simulink model "gm_HDLQAMDemod_vs"  (R2024a)
settings: Solver=FixedStepDiscrete  StartTime=0.0  StopTime=stopTime  RelTol=1e-3
undefined symbols (not defined in the file or in its folder): clk, clk_enable, fs, QAM, reset_x
libraries: dspsrcs4 x3, whdlmod x3, simulink x2, whdlutilities x1, vivadosimlib x1, HDL_ieee_8021513 x1
settings Model: Creator=cotti  LastModifiedBy=cotti
settings OptimizationCC: BlockReduction=off  ConditionallyExecuteInputs=off  DefaultParameterBehavior=Inlined  InheritOutputTypeSmallerThanSingle=on
settings DebuggingCC: AlgebraicLoopMsg=error  ArtificialAlgebraicLoopMsg=error  InheritedTsInSrcMsg=none  SingleTaskRateTransMsg=error  UnconnectedInputMsg=warning  UnconnectedOutputMsg=warning  UnconnectedLineMsg=warning
settings HardwareCC: ProdBitPerPointer=32  ProdBitPerSizeT=32  ProdBitPerPtrDiffT=32  ProdLargestAtomicFloat=None  ProdIntDivRoundTo=Undefined  ProdEndianess=Unspecified  ProdWordSize=32  ProdHWDeviceType=ASIC/FPGA->ASIC/FPGA  TargetBitPerLong=64  TargetBitPerPointer=64  TargetBitPerSizeT=64  TargetBitPerPtrDiffT=64  TargetLongLongMode=on  TargetIntDivRoundTo=Zero  TargetEndianess=LittleEndian  TargetWordSize=64  TargetHWDeviceType=Custom Processor->MATLAB Host Computer  ProdEqTarget=off

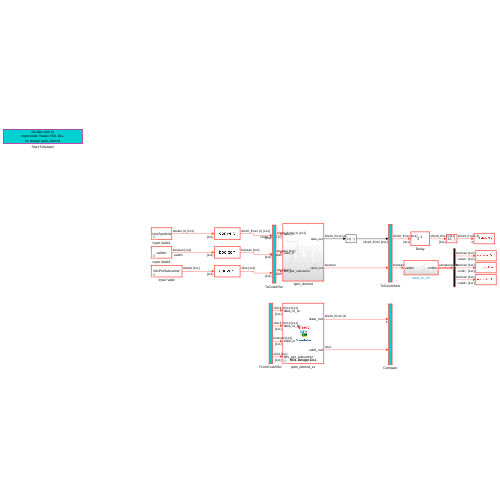
[thumbnail: Simulink's stored preview of the top-level diagram]
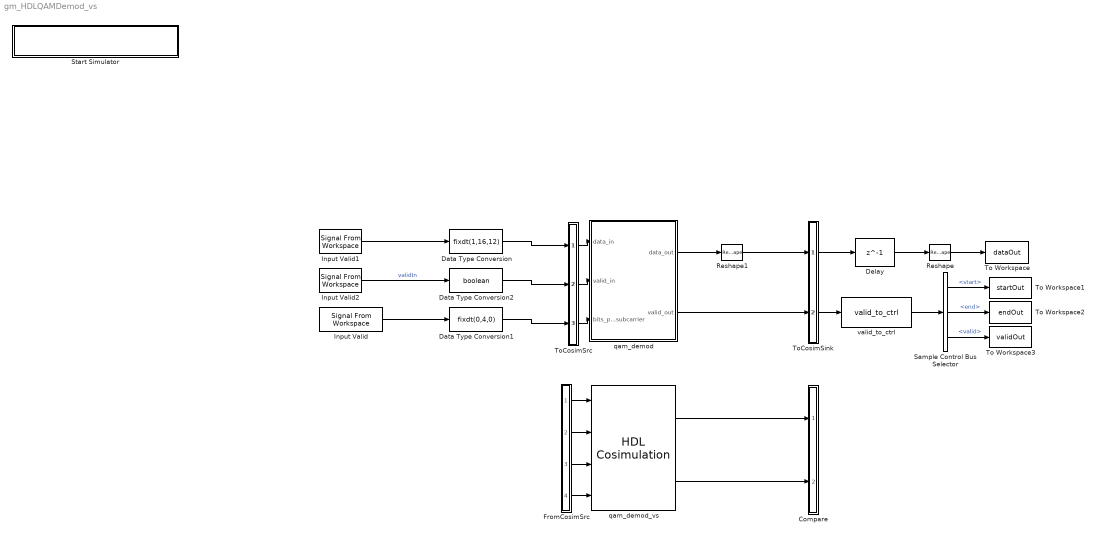
== system gm_HDLQAMDemod_vs ==
  Compare : Subsystem
      mask Display: disp('')
  Data Type Conversion : DataTypeConversion  OutDataTypeStr=fixdt(1,16,12)  SaturateOnIntegerOverflow=off  RndMeth=Floor
  Data Type Conversion1 : DataTypeConversion  OutDataTypeStr=fixdt(0,4,0)  SaturateOnIntegerOverflow=off  RndMeth=Floor
  Data Type Conversion2 : DataTypeConversion  OutDataTypeStr=boolean  SaturateOnIntegerOverflow=off  RndMeth=Floor
  Delay : Delay  DelayLength=1  InitialCondition=0  UseCircularBuffer=on
  FromCosimSrc : Subsystem
      mask Display: disp('')
  Input Valid : dspsrcs4/Signal From Workspace  X=bitsPerSubcarrier  Ts=1/fs  nsamps=1  OutputAfterFinalValue=Setting to zero  ignoreOrWarnInputAndFrameLengths=off  OutputFrames=off
  Input Valid1 : dspsrcs4/Signal From Workspace  X=dataSymbols  Ts=1/fs  nsamps=1  OutputAfterFinalValue=Setting to zero  ignoreOrWarnInputAndFrameLengths=off  OutputFrames=off
  Input Valid2 : dspsrcs4/Signal From Workspace  X=validIn  Ts=1/fs  nsamps=1  OutputAfterFinalValue=Setting to zero  ignoreOrWarnInputAndFrameLengths=off  OutputFrames=off
  Reshape : Reshape
  Reshape1 : Reshape
  Sample Control Bus Selector : whdlutilities/Sample Control Bus Selector  OutputSignals=start,end,valid
  Start Simulator : Subsystem
      settings: OpenFcn=|
      | cosimDirName = pwd;
      | cd 'hdl_prj/hdlsrc/HDLQAMDemod';
      | [s,r] = system('vivado -mode batch -source gm_HDLQAMDemod_vs.tcl','-echo');
      | cd (cosimDirName);
      | clear cosimDirName;
      | if s
      |    error('Failed to create Vivado HDL design DLL using script gm_HDLQAMDemod_vs.tcl.');
      | end
      mask Display: disp('Double-click to\nregenerate Vivado HDL DLL\nfor design qam_demod')
  To Workspace : ToWorkspace  VariableName=dataOut  SampleTime=1/fs
      settings: Save2DSignal=2-D array (concatenate along first dimension)
  To Workspace1 : ToWorkspace  VariableName=startOut  SampleTime=1/fs
      settings: Save2DSignal=2-D array (concatenate along first dimension)
  To Workspace2 : ToWorkspace  VariableName=endOut  SampleTime=1/fs
      settings: Save2DSignal=2-D array (concatenate along first dimension)
  To Workspace3 : ToWorkspace  VariableName=validOut  SampleTime=1/fs
      settings: Save2DSignal=2-D array (concatenate along first dimension)
  ToCosimSink : Subsystem
      mask Display: disp('')
  ToCosimSrc : Subsystem
      mask Display: disp('')
  qam_demod : Subsystem
  qam_demod_vs : vivadosimlib/HDL Cosimulation  PortPaths=/qam_demod/data_in_re;/qam_demod/data_in_im;/qam_demod/valid_in;/qam_demod/bits_per_subcarrier;/qam_demod/data_out;/qam_demod/valid_out  PortModes=[1 1 1 1 2 2 ]  PortTimes=[-1 -1 -1 -1 1.0000000000000000209225608301284726753266340892878361046314239502e-08 1.0000000000000000209225608301284726753266340892878361046314239502e-08 ]  PortSigns=[-1 -1 -1 -1 1 0 ]  PortFracLengths=[0,0,0,0,12,0]  PortWordLengths=[-1,-1,-1,-1,20,1]  PortHDLWordSizes=[16,16,1,4,20,1]  CommLocal=on  CommSharedMemory=on  CommPortNumber=4449  CommShowInfo=on  ClockPaths=clk;clk_enable;reset_x;  ClockModes=[2 4 3]  ClockTimes=[1e-08 3.7e-08 2.7e-08]  TclPostSimCommand="puts \"done\""  TimingMode=ns  TimingScaleFactor=1000000000  idxCellArray={'UNUSED_VAR'}  CosimBypass=Full Simulation  AllowDirectFeedthrough=on  ProductName=EDA Simulator Link VS  RunAutoTimescale=off  HdlClocks=0  PreRunTime=40  PreRunTimeUnit=ns
  valid_to_ctrl : HDL_ieee_8021513/valid_to_ctrl  SystemSampleTime=-1  VariantActivationTime=update diagram  AllowFlexibleInterface=on  Latency=0  AutoFrameSizeCalculation=off
      settings: SourceProductName=HDL IEEE 8021513
  wires:
  Sample Control Bus Selector/2 -> To Workspace2/1  "<end>"
  Input Valid/1 -> Data Type Conversion1/1
  Input Valid2/1 -> Data Type Conversion2/1  "validIn"
  Sample Control Bus Selector/3 -> To Workspace3/1  "<valid>"
  Input Valid1/1 -> Data Type Conversion/1
  valid_to_ctrl/1 -> Sample Control Bus Selector/1
  Sample Control Bus Selector/1 -> To Workspace1/1  "<start>"
  Delay/1 -> Reshape/1
  Reshape/1 -> To Workspace/1
  ToCosimSrc/1(out1) -> qam_demod/1(data_in)
  ToCosimSrc/2(out2) -> qam_demod/2(valid_in)
  ToCosimSrc/3(out3) -> qam_demod/3(bits_per_subcarrier)
  qam_demod/1(data_out) -> Reshape1/1
  qam_demod/2(valid_out) -> ToCosimSink/2(in2)
  Data Type Conversion/1 -> ToCosimSrc/1(in1)
  Data Type Conversion2/1 -> ToCosimSrc/2(in2)
  Data Type Conversion1/1 -> ToCosimSrc/3(in3)
  ToCosimSink/1(out1) -> Delay/1
  ToCosimSink/2(out2) -> valid_to_ctrl/1
  FromCosimSrc/1(out1) -> qam_demod_vs/1
  FromCosimSrc/2(out2) -> qam_demod_vs/2
  FromCosimSrc/3(out3) -> qam_demod_vs/3
  FromCosimSrc/4(out4) -> qam_demod_vs/4
  qam_demod_vs/1 -> Compare/1(in1)
  qam_demod_vs/2 -> Compare/2(in2)
  Reshape1/1 -> ToCosimSink/1(in1)

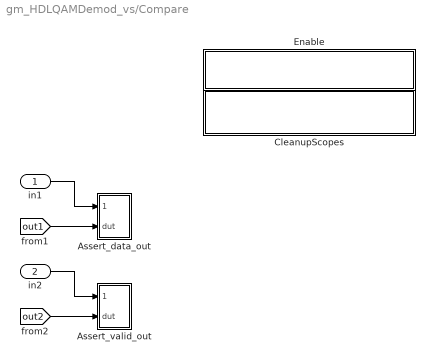
== system gm_HDLQAMDemod_vs/Compare ==
  in1 : Inport
  in2 : Inport  Port=2
  Assert_data_out : Subsystem
      settings: LibrarySourceBlock=hdlmdlgenlib/AssertEq
  Assert_valid_out : Subsystem
      settings: LibrarySourceBlock=hdlmdlgenlib/AssertEq
  CleanupScopes : Subsystem
      settings: OpenFcn=|
      | blkName = gcb; %self block
      | idx = regexp(blkName, '/CleanupScopes$', 'once');
      | blkParent = blkName(1:idx-1);
      | blks=find_system(blkParent, 'LookUnderMasks', 'all','blocktype', 'Scope');
      | for itr = 1:length(blks)
      | 	 hScopeCfg = get_param(blks{itr},'ScopeConfiguration');
      | 	 hScopeCfg.Visible = ~ hScopeCfg.Visible;
      | end
      | drawnow;
      mask Display: fprintf(message('hdlcoder:cosim:vnl_dblclick').getString());
  Enable : Subsystem
      settings: OpenFcn=|
      | blkName = gcb;
      | idx = regexp(blkName, '/Enable$', 'once');
      | blkParent = blkName(1:idx-1);
      | blks=find_system(blkParent, 'LookUnderMasks', 'all','blocktype', 'Assertion');
      | e = get_param(blks{1}, 'Enabled');
      | if strcmp(e, 'on'), f= 'off';, else, f = 'on';, end
      | for ii=1:length(blks), set_param(blks{ii}, 'Enabled', f);, end
      | set_param(gcb, 'MaskDisplay',['fprintf(message(''hdlcoder:cosim:vnl_dblclick_assertions'',','''',upper(e),'''',').getString())']);
      mask Display: fprintf(message('hdlcoder:cosim:vnl_dblclick_assertions','OFF').getString());
  wires:
  [out2] -> Assert_valid_out/2(dut)
  in2/1 -> Assert_valid_out/1(cosim)
  [out1] -> Assert_data_out/2(dut)
  in1/1 -> Assert_data_out/1(cosim)

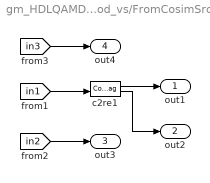
== system gm_HDLQAMDemod_vs/FromCosimSrc ==
  c2re1 : ComplexToRealImag
  out1 : Outport
  out2 : Outport  Port=2
  out3 : Outport  Port=3
  out4 : Outport  Port=4
  wires:
  c2re1/2 -> out2/1
  [in2] -> out3/1
  [in1] -> c2re1/1
  c2re1/1 -> out1/1
  [in3] -> out4/1

== system gm_HDLQAMDemod_vs/Start Simulator ==

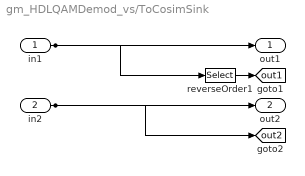
== system gm_HDLQAMDemod_vs/ToCosimSink ==
  in1 : Inport
  in2 : Inport  Port=2
  reverseOrder1 : Selector  IndexOptions=Index vector (dialog)  Indices=[4:-1:1]  OutputSizes=1
  out1 : Outport
  out2 : Outport  Port=2
  tag scope: out1=global, out2=global
  wires:
  in1/1 -> out1/1, reverseOrder1/1
  reverseOrder1/1 -> [out1]
  in2/1 -> out2/1, [out2]

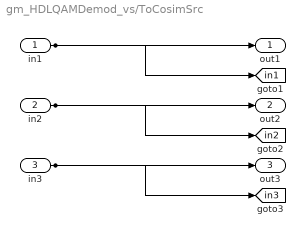
== system gm_HDLQAMDemod_vs/ToCosimSrc ==
  in1 : Inport
  in2 : Inport  Port=2
  in3 : Inport  Port=3
  out1 : Outport
  out2 : Outport  Port=2
  out3 : Outport  Port=3
  tag scope: in1=global, in2=global, in3=global
  wires:
  in1/1 -> out1/1, [in1]
  in2/1 -> out2/1, [in2]
  in3/1 -> out3/1, [in3]

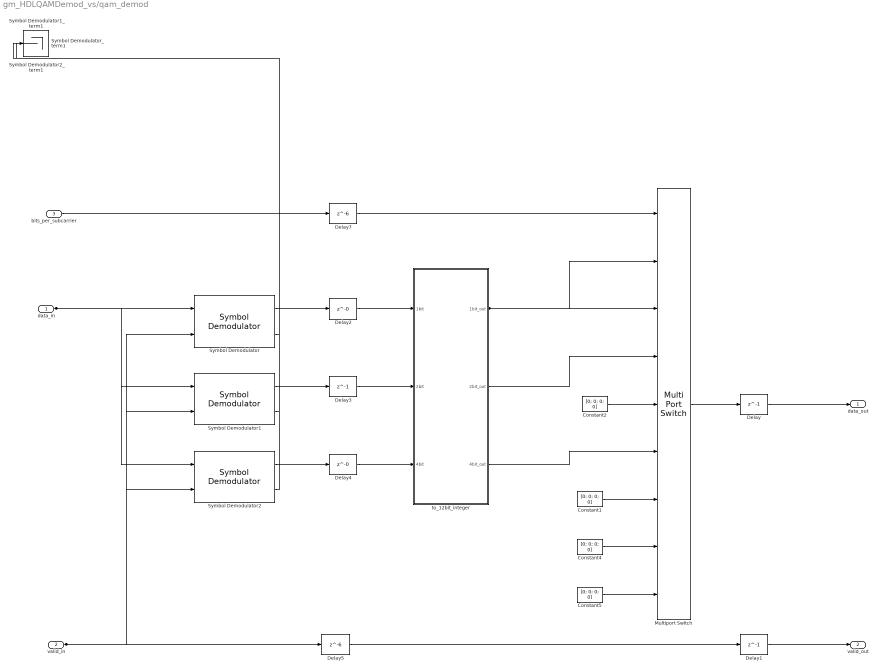
== system gm_HDLQAMDemod_vs/qam_demod ==
  data_in : Inport  OutDataTypeStr=fixdt(1, 16, 12)  PortDimensions=1  SampleTime=1e-08
      settings: SignalType=complex
  valid_in : Inport  Port=2  OutDataTypeStr=boolean  PortDimensions=1  SampleTime=1e-08
  bits_per_subcarrier : Inport  Port=3  OutDataTypeStr=fixdt(0, 4, 0)  PortDimensions=1  SampleTime=1e-08
  Constant{1..2,4..5} (4 alike) : Constant  Value=[0; 0; 0; 0]  VectorParams1D=off  OutDataTypeStr=fixdt(1, 20, 12)  SampleTime=-1  LockScale=on
  Delay : Delay  DelayLength=1  InitialCondition=0  UseCircularBuffer=on
  Delay1 : Delay  DelayLength=1  InitialCondition=0  UseCircularBuffer=on
  Delay2 : Delay  DelayLength=0  InitialCondition=0  UseCircularBuffer=on
  Delay3 : Delay  DelayLength=1  InitialCondition=0  UseCircularBuffer=on
  Delay4 : Delay  DelayLength=0  InitialCondition=0  UseCircularBuffer=on
  Delay5 : Delay  DelayLength=6  InitialCondition=0  UseCircularBuffer=on
  Delay7 : Delay  DelayLength=6  InitialCondition=0  UseCircularBuffer=on
  Multiport Switch : MultiPortSwitch  DataPortOrder=Zero-based contiguous  Inputs=8  zeroidx=on  OutDataTypeStr=fixdt(1, 20, 12)  SaturateOnIntegerOverflow=off
  Symbol Demodulator : whdlmod/Symbol Demodulator  ModulationSource=Property  ModulationScheme=BPSK  MaxModulation=256-QAM  ConstOrder=Default  ConstMap=[ 2, 3, 1, 0, 6, 7, 5, 4, 14, 15, 13, 12, 10, 11, 9, 8 ]  DecisionType=Approximate log-likelihood ratio  PhaseOffset=0  OutputType=Vector  NormMethod=Unit average power  MinSymDistance=2  NoiseVariance=off  SimulateUsing=Code generation
  Symbol Demodulator1 : whdlmod/Symbol Demodulator  ModulationSource=Property  ModulationScheme=QPSK  MaxModulation=256-QAM  ConstOrder=Default  ConstMap=[ 2, 3, 1, 0, 6, 7, 5, 4, 14, 15, 13, 12, 10, 11, 9, 8 ]  DecisionType=Approximate log-likelihood ratio  PhaseOffset=-pi/4  OutputType=Vector  NormMethod=Unit average power  MinSymDistance=2  NoiseVariance=off  SimulateUsing=Code generation
  Symbol Demodulator1_term1 : Terminator
  Symbol Demodulator2 : whdlmod/Symbol Demodulator  ModulationSource=Property  ModulationScheme=16-QAM  MaxModulation=256-QAM  ConstOrder=Default  ConstMap=qamFourBits.'  DecisionType=Approximate log-likelihood ratio  PhaseOffset=pi/2  OutputType=Vector  NormMethod=Unit average power  MinSymDistance=2  NoiseVariance=off  SimulateUsing=Code generation
  Symbol Demodulator2_term1 : Terminator
  Symbol Demodulator_term1 : Terminator
  to_12bit_integer : Subsystem
  data_out : Outport  SampleTime=1e-08
  valid_out : Outport  Port=2  SampleTime=1e-08  VectorParamsAs1DForOutWhenUnconnected=off
  wires:
  to_12bit_integer/3(4bit_out) -> Multiport Switch/6
  to_12bit_integer/2(2bit_out) -> Multiport Switch/4
  to_12bit_integer/1(1bit_out) -> Multiport Switch/2, Multiport Switch/3
  Symbol Demodulator2/2 -> Symbol Demodulator2_term1/1
  Symbol Demodulator2/1 -> Delay4/1
  Symbol Demodulator1/2 -> Symbol Demodulator1_term1/1
  Symbol Demodulator1/1 -> Delay3/1
  Symbol Demodulator/2 -> Symbol Demodulator_term1/1
  Symbol Demodulator/1 -> Delay2/1
  Multiport Switch/1 -> Delay/1
  Delay7/1 -> Multiport Switch/1
  Delay5/1 -> Delay1/1
  Delay4/1 -> to_12bit_integer/3(4bit)
  Delay3/1 -> to_12bit_integer/2(2bit)
  Delay2/1 -> to_12bit_integer/1(1bit)
  Delay1/1 -> valid_out/1
  Delay/1 -> data_out/1
  Constant5/1 -> Multiport Switch/9
  Constant4/1 -> Multiport Switch/8
  Constant2/1 -> Multiport Switch/5
  Constant1/1 -> Multiport Switch/7
  bits_per_subcarrier/1 -> Delay7/1
  valid_in/1 -> Symbol Demodulator2/2, Symbol Demodulator1/2, Symbol Demodulator/2, Delay5/1
  data_in/1 -> Symbol Demodulator2/1, Symbol Demodulator1/1, Symbol Demodulator/1

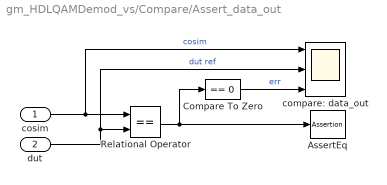
== system gm_HDLQAMDemod_vs/Compare/Assert_data_out ==
  cosim : Inport
  dut : Inport  Port=2
  AssertEq : Assertion
  Compare To Zero : simulink/Logic and Bit Operations/Compare To Zero  relop===  OutDataTypeStr=boolean
  Relational Operator : RelationalOperator  Operator===  OutDataTypeStr=boolean  InputSameDT=off
  compare: data_out : Scope  NumInputPorts=3
  wires:
  Compare To Zero/1 -> compare: data_out/3  "err"
  Relational Operator/1 -> Compare To Zero/1, AssertEq/1
  cosim/1 -> compare: data_out/1, Relational Operator/1  "cosim"
  dut/1 -> compare: data_out/2, Relational Operator/2  "dut ref"

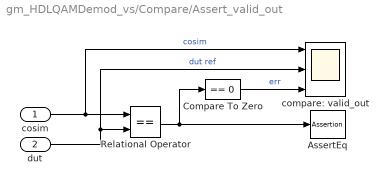
== system gm_HDLQAMDemod_vs/Compare/Assert_valid_out ==
  cosim : Inport
  dut : Inport  Port=2
  AssertEq : Assertion
  Compare To Zero : simulink/Logic and Bit Operations/Compare To Zero  relop===  OutDataTypeStr=boolean
  Relational Operator : RelationalOperator  Operator===  OutDataTypeStr=boolean  InputSameDT=off
  compare: valid_out : Scope  NumInputPorts=3
  wires:
  Compare To Zero/1 -> compare: valid_out/3  "err"
  Relational Operator/1 -> Compare To Zero/1, AssertEq/1
  cosim/1 -> compare: valid_out/1, Relational Operator/1  "cosim"
  dut/1 -> compare: valid_out/2, Relational Operator/2  "dut ref"

== system gm_HDLQAMDemod_vs/Compare/CleanupScopes ==

== system gm_HDLQAMDemod_vs/Compare/Enable ==

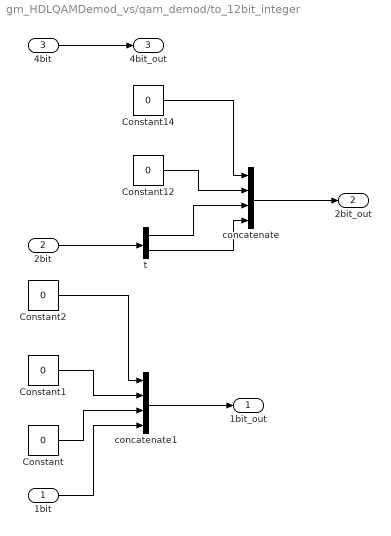
== system gm_HDLQAMDemod_vs/qam_demod/to_12bit_integer ==
  1bit : Inport  OutDataTypeStr=fixdt(1, 20, 12)  PortDimensions=1  SampleTime=1e-08
  2bit : Inport  Port=2  OutDataTypeStr=fixdt(1, 20, 12)  PortDimensions=[2 1]  SampleTime=1e-08
  4bit : Inport  Port=3  OutDataTypeStr=fixdt(1, 20, 12)  PortDimensions=[4 1]  SampleTime=1e-08
  Constant{,1..2,12,14} (5 alike) : Constant  Value=0  OutDataTypeStr=fixdt(1, 20, 12)  SampleTime=1e-08
  concatenate : Concatenate  NumInputs=4  Mode=Multidimensional array
  concatenate1 : Concatenate  NumInputs=4  Mode=Multidimensional array
  t : Demux  Outputs=2
  1bit_out : Outport  SampleTime=1e-08
  2bit_out : Outport  Port=2  SampleTime=1e-08
  4bit_out : Outport  Port=3  SampleTime=1e-08
  wires:
  t/2 -> concatenate/4
  t/1 -> concatenate/3
  concatenate1/1 -> 1bit_out/1
  concatenate/1 -> 2bit_out/1
  Constant2/1 -> concatenate1/1
  Constant14/1 -> concatenate/1
  Constant12/1 -> concatenate/2
  Constant1/1 -> concatenate1/2
  Constant/1 -> concatenate1/3
  4bit/1 -> 4bit_out/1
  2bit/1 -> t/1
  1bit/1 -> concatenate1/4
